simulink model "Smart_Inverter_IEEE33_Results_Viewer"  (R2026a)
settings: Solver=FixedStepDiscrete  StopTime=23  FixedStep=1
InitFcn:
  | startup_project; prepare_simulink_visualization_data('stress_100pct_clear_low_daytime','hybrid_pso');
settings Model: Creator=ismahin  LastModifiedBy=ismahin

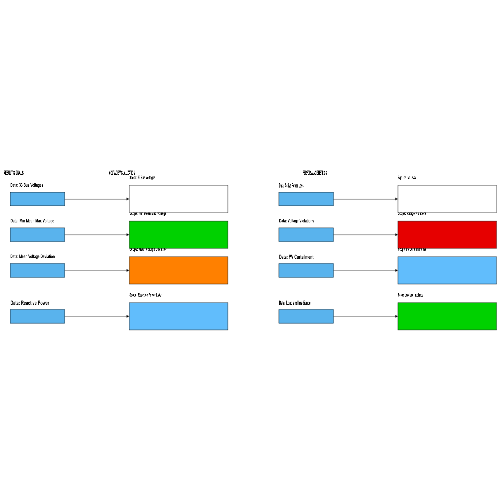
[thumbnail: Simulink's stored preview of the top-level diagram]
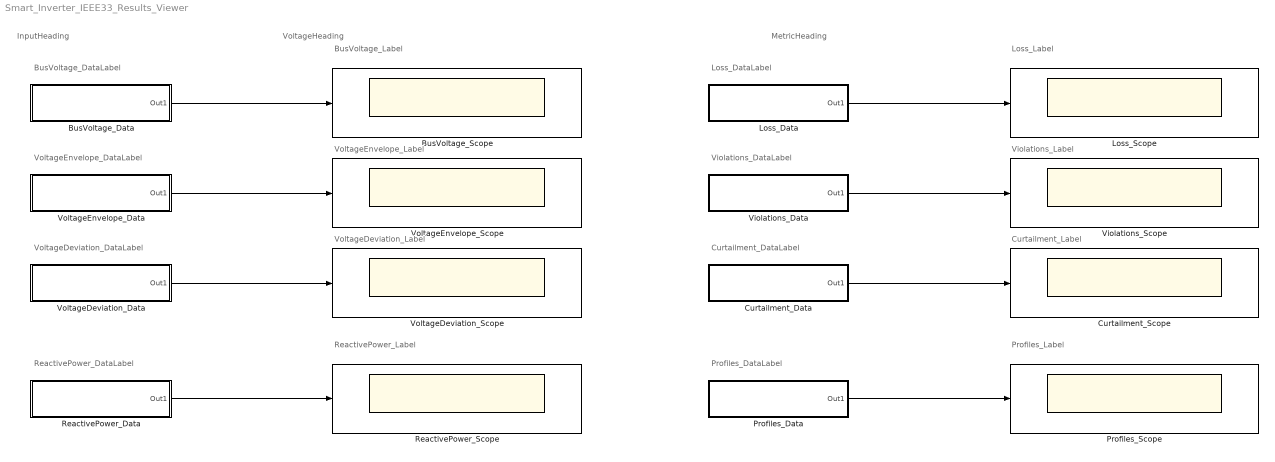
== system Smart_Inverter_IEEE33_Results_Viewer ==
  note: InputHeading
  note: VoltageHeading
  note: MetricHeading
  note: BusVoltage_DataLabel
  note: BusVoltage_Label
  note: VoltageEnvelope_DataLabel
  note: VoltageEnvelope_Label
  note: VoltageDeviation_DataLabel
  note: VoltageDeviation_Label
  note: Loss_DataLabel
  note: Loss_Label
  note: Violations_DataLabel
  note: Violations_Label
  note: Curtailment_DataLabel
  note: Curtailment_Label
  note: ReactivePower_DataLabel
  note: ReactivePower_Label
  note: Profiles_DataLabel
  note: Profiles_Label
  BusVoltage_Data : Subsystem
      mask Display: color('blue'); patch([0 1 1 0],[0 0 1 1],[0.35 0.70 0.93]);
  BusVoltage_Scope : Scope
  Curtailment_Data : Subsystem
      mask Display: color('blue'); patch([0 1 1 0],[0 0 1 1],[0.35 0.70 0.93]);
  Curtailment_Scope : Scope
  Loss_Data : Subsystem
      mask Display: color('blue'); patch([0 1 1 0],[0 0 1 1],[0.35 0.70 0.93]);
  Loss_Scope : Scope
  Profiles_Data : Subsystem
      mask Display: color('blue'); patch([0 1 1 0],[0 0 1 1],[0.35 0.70 0.93]);
  Profiles_Scope : Scope
  ReactivePower_Data : Subsystem
      mask Display: color('blue'); patch([0 1 1 0],[0 0 1 1],[0.35 0.70 0.93]);
  ReactivePower_Scope : Scope
  Violations_Data : Subsystem
      mask Display: color('blue'); patch([0 1 1 0],[0 0 1 1],[0.35 0.70 0.93]);
  Violations_Scope : Scope
  VoltageDeviation_Data : Subsystem
      mask Display: color('blue'); patch([0 1 1 0],[0 0 1 1],[0.35 0.70 0.93]);
  VoltageDeviation_Scope : Scope
  VoltageEnvelope_Data : Subsystem
      mask Display: color('blue'); patch([0 1 1 0],[0 0 1 1],[0.35 0.70 0.93]);
  VoltageEnvelope_Scope : Scope
  wires:
  BusVoltage_Data/1(Out1) -> BusVoltage_Scope/1
  VoltageEnvelope_Data/1(Out1) -> VoltageEnvelope_Scope/1
  VoltageDeviation_Data/1(Out1) -> VoltageDeviation_Scope/1
  Loss_Data/1(Out1) -> Loss_Scope/1
  Violations_Data/1(Out1) -> Violations_Scope/1
  Curtailment_Data/1(Out1) -> Curtailment_Scope/1
  ReactivePower_Data/1(Out1) -> ReactivePower_Scope/1
  Profiles_Data/1(Out1) -> Profiles_Scope/1

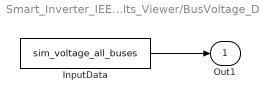
== system Smart_Inverter_IEEE33_Results_Viewer/BusVoltage_Data ==
  InputData : FromWorkspace  VariableName=sim_voltage_all_buses
  Out1 : Outport
  wires:
  InputData/1 -> Out1/1

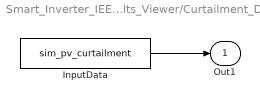
== system Smart_Inverter_IEEE33_Results_Viewer/Curtailment_Data ==
  InputData : FromWorkspace  VariableName=sim_pv_curtailment
  Out1 : Outport
  wires:
  InputData/1 -> Out1/1

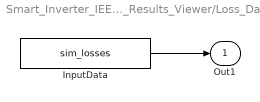
== system Smart_Inverter_IEEE33_Results_Viewer/Loss_Data ==
  InputData : FromWorkspace  VariableName=sim_losses
  Out1 : Outport
  wires:
  InputData/1 -> Out1/1

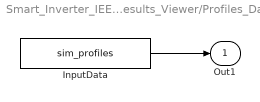
== system Smart_Inverter_IEEE33_Results_Viewer/Profiles_Data ==
  InputData : FromWorkspace  VariableName=sim_profiles
  Out1 : Outport
  wires:
  InputData/1 -> Out1/1

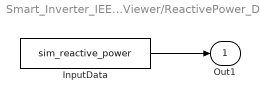
== system Smart_Inverter_IEEE33_Results_Viewer/ReactivePower_Data ==
  InputData : FromWorkspace  VariableName=sim_reactive_power
  Out1 : Outport
  wires:
  InputData/1 -> Out1/1

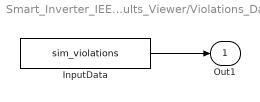
== system Smart_Inverter_IEEE33_Results_Viewer/Violations_Data ==
  InputData : FromWorkspace  VariableName=sim_violations
  Out1 : Outport
  wires:
  InputData/1 -> Out1/1

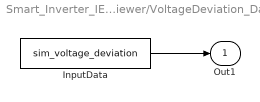
== system Smart_Inverter_IEEE33_Results_Viewer/VoltageDeviation_Data ==
  InputData : FromWorkspace  VariableName=sim_voltage_deviation
  Out1 : Outport
  wires:
  InputData/1 -> Out1/1

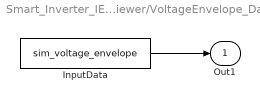
== system Smart_Inverter_IEEE33_Results_Viewer/VoltageEnvelope_Data ==
  InputData : FromWorkspace  VariableName=sim_voltage_envelope
  Out1 : Outport
  wires:
  InputData/1 -> Out1/1
